simulink model "pidctrl_modelR2011a"  (Simulink 7.7)
settings: Solver=ode15s  StartTime=0.0  StopTime=10.0  MaxStep=1000  RelTol=1e-5
values from neighbouring files (symbols this model uses):
  Kd = 1.73855406815    [IAE.mat]
  keyCriterion = 3    [IAE.mat]
  Ki = 0.608530675407    [IAE.mat]
  Kp = 1.83556226215    [IAE.mat]
libraries: simulink x1
settings Model: Creator=Professor Dingyu Xue  LastModifiedBy=Professor Dingyu Xue
settings SolverCC: ZeroCrossControl=DisableAll
settings DataIOCC: LimitDataPoints=off
settings DebuggingCC: SolverPrmCheckMsg=none

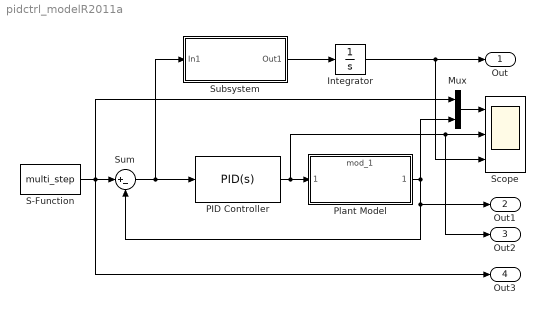
== system pidctrl_modelR2011a ==
  Integrator : Integrator
  Mux : Mux  Inputs=2
  PID Controller : simulink/Continuous/PID Controller  SystemSampleTime=-1  Controller=PID  TimeDomain=Continuous-time  SampleTime=1  IntegratorMethod=Forward Euler  FilterMethod=Forward Euler  Form=Parallel  P=Kp  I=Ki  D=Kd  N=100  InitialConditionSource=internal  InitialConditionForIntegrator=0  InitialConditionForFilter=0  ExternalReset=none  LimitOutput=off  UpperSaturationLimit=inf  LowerSaturationLimit=-inf  LinearizeAsGain=off  AntiWindupMode=none  Kb=1  TrackingMode=off  Kt=1  PParamMin=[]  PParamMax=[]  IParamMin=[]  IParamMax=[]  DParamMin=[]  DParamMax=[]  NParamMin=[]  NParamMax=[]  KbParamMin=[]  KbParamMax=[]  KtParamMin=[]  KtParamMax=[]  POutMin=[]  POutMax=[]  IOutMin=[]  IOutMax=[]  DOutMin=[]  DOutMax=[]  NOutMin=[]  NOutMax=[]  KbOutMin=[]  KbOutMax=[]  KtOutMin=[]  KtOutMax=[]  IntegratorOutMin=[]  IntegratorOutMax=[]  FilterOutMin=[]  FilterOutMax=[]  SumOutMin=[]  SumOutMax=[]  SumI1OutMin=[]  SumI1OutMax=[]  SumI2OutMin=[]  SumI2OutMax=[]  SumI3OutMin=[]  SumI3OutMax=[]  SumDOutMin=[]  SumDOutMax=[]  SaturationOutMin=[]  SaturationOutMax=[]  IntegratorContinuousStateAttributes=''  IntegratorStateMustResolveToSignalObject=off  IntegratorRTWStateStorageClass=Auto  FilterContinuousStateAttributes=''  FilterStateMustResolveToSignalObject=off  FilterRTWStateStorageClass=Auto
  Plant Model : ModelReference  ModelNameDialog=mod_1  SimulationMode=Normal  ModelReferenceVersion=1.4  CopyOfModelName=mod_1  DefaultDataLogging=on
  S-Function : S-Function  FunctionName=multi_step  Parameters=t_seq, y_seq  EnableBusSupport=off
  Scope : Scope  NumInputPorts=3
      settings: YMin=0~0~0  YMax=1.5~40~1.5  SaveName=yy
  Subsystem : Subsystem
  Sum : Sum  Inputs=|+-
  Out : Outport
  Out1 : Outport  Port=2
  Out2 : Outport  Port=3
  Out3 : Outport  Port=4
  wires:
  Sum/1 -> PID Controller/1, Subsystem/1(In1)
  S-Function/1 -> Sum/1, Mux/1, Out3/1
  PID Controller/1 -> Plant Model/1, Scope/2, Out2/1
  Plant Model/1 -> Mux/2, Sum/2, Out1/1
  Mux/1 -> Scope/1
  Subsystem/1(Out1) -> Integrator/1
  Integrator/1 -> Out/1, Scope/3

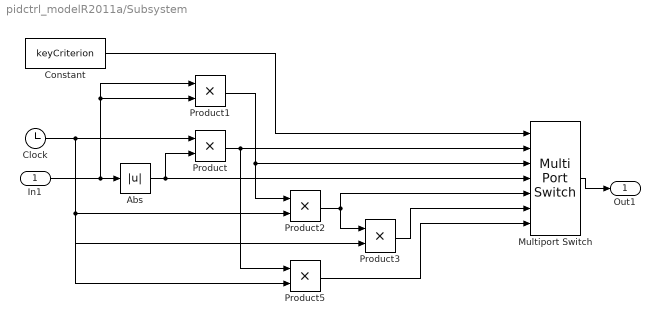
== system pidctrl_modelR2011a/Subsystem ==
  In1 : Inport
  Abs : Abs
  Clock : Clock
      settings: Decimation=10
  Constant : Constant  Value=keyCriterion
  Multiport Switch : MultiPortSwitch  Inputs=6  zeroidx=off
  Product{,1..3,5} (5 alike) : Product  RndMeth=Zero
  Out1 : Outport
  wires:
  Constant/1 -> Multiport Switch/1
  Product1/1 -> Multiport Switch/3, Product2/1
  Product/1 -> Product5/1, Multiport Switch/2
  Clock/1 -> Product/1, Product2/2, Product3/2, Product5/2
  In1/1 -> Product1/2, Product1/1, Abs/1
  Abs/1 -> Product/2, Multiport Switch/4
  Multiport Switch/1 -> Out1/1
  Product2/1 -> Multiport Switch/5, Product3/1
  Product3/1 -> Multiport Switch/6
  Product5/1 -> Multiport Switch/7
